simulink model "p1"  (R2021b)
settings: Solver=VariableStepAuto  StartTime=0.0  StopTime=30  RelTol=1e-3
libraries: simulink x2
settings Model: Creator=hp  LastModifiedBy=hp

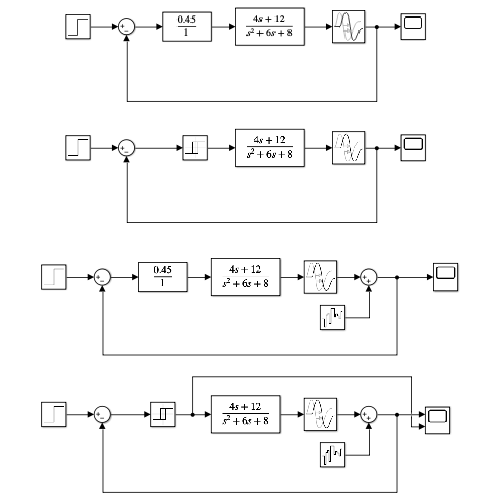
[thumbnail: Simulink's stored preview of the top-level diagram]
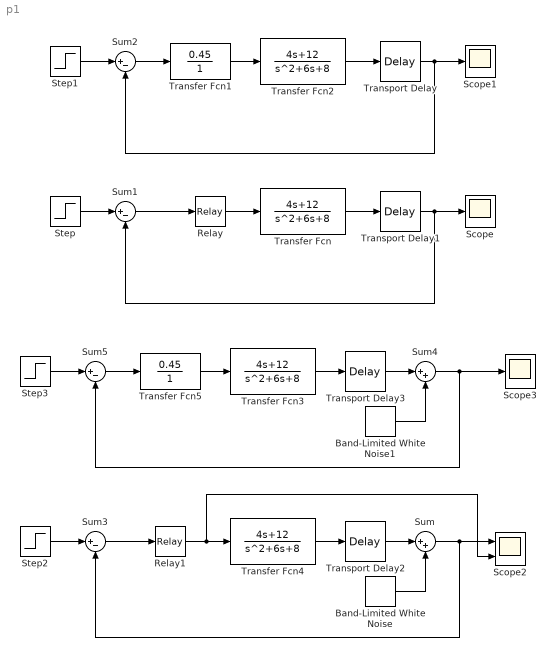
== system p1 ==
  Band-Limited White Noise : simulink/Sources/Band-Limited White Noise  Cov=[0.1]  Ts=0.1  seed=[23341]
  Band-Limited White Noise1 : simulink/Sources/Band-Limited White Noise  Cov=[0.1]  Ts=0.1  seed=[23341]
  Relay : Relay  OnOutputValue=0.45  OffOutputValue=-0.45
  Relay1 : Relay  OnSwitchValue=1  OffSwitchValue=-1  OnOutputValue=2  OffOutputValue=-2
  Scope : Scope
  Scope1 : Scope
  Scope2 : Scope  NumInputPorts=2
  Scope3 : Scope
  Step{,1..3} (4 alike) : Step  SampleTime=0
  Sum : Sum  Inputs=|++
  Sum{1..3,5} (4 alike) : Sum  Inputs=|+-
  Sum4 : Sum  Inputs=|++
  Transfer Fcn{,2..4} (4 alike) : TransferFcn  Numerator=[4 12]  Denominator=[1 6 8]
  Transfer Fcn1 : TransferFcn  Numerator=[0.45]  Denominator=[1]
  Transfer Fcn5 : TransferFcn  Numerator=[0.45]  Denominator=[1]
  Transport Delay{,1..3} (4 alike) : TransportDelay
  wires:
  Transfer Fcn/1 -> Transport Delay1/1
  Relay/1 -> Transfer Fcn/1
  Sum1/1 -> Relay/1
  Step/1 -> Sum1/1
  Transport Delay1/1 -> Sum1/2, Scope/1
  Step1/1 -> Sum2/1
  Transport Delay/1 -> Sum2/2, Scope1/1
  Transfer Fcn2/1 -> Transport Delay/1
  Transfer Fcn1/1 -> Transfer Fcn2/1
  Sum2/1 -> Transfer Fcn1/1
  Sum3/1 -> Relay1/1
  Transfer Fcn4/1 -> Transport Delay2/1
  Step2/1 -> Sum3/1
  Transport Delay2/1 -> Sum/1
  Sum/1 -> Sum3/2, Scope2/1
  Band-Limited White Noise/1 -> Sum/2
  Relay1/1 -> Scope2/2, Transfer Fcn4/1
  Band-Limited White Noise1/1 -> Sum4/2
  Transport Delay3/1 -> Sum4/1
  Step3/1 -> Sum5/1
  Transfer Fcn3/1 -> Transport Delay3/1
  Sum4/1 -> Sum5/2, Scope3/1
  Transfer Fcn5/1 -> Transfer Fcn3/1
  Sum5/1 -> Transfer Fcn5/1
